simulink model "same_v2"  (R2014b)
settings: Solver=ode45  StartTime=0  StopTime=5  RelTol=1e-3
values from neighbouring files (symbols this model uses):
  a_11 = (a^2*k_1+b^2*k_2)/I_z/u    (= -24.3328872171)    [model.m]
  a_12 = (a*k_1-b*k_2)/I_z    (= 2.49734914361)    [model.m]
  a_21 = (a*k_1-b*k_2)/m/u^2-1    (= -0.900945465806)    [model.m]
  a_22 = (k_1+k_2)/m/u    (= -18.4476774194)    [model.m]
  b_11 = -a*k_1/I_z    (= 50.9018603426)    [model.m]
  b_21 = -k_1/m/u    (= 10.8267096774)    [model.m]
settings Model: Creator=暖的一笔的大学生  LastModifiedBy=暖的一笔的大学生

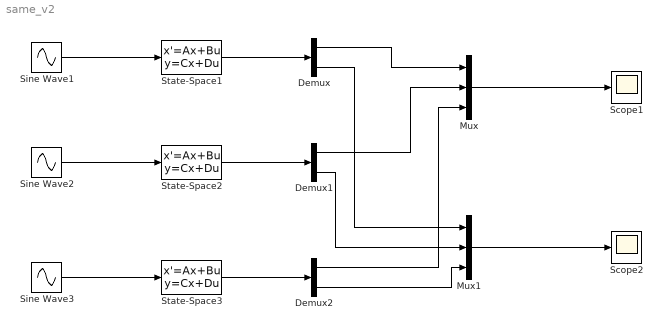
== system same_v2 ==
  Demux : Demux  Outputs=2
  Demux1 : Demux  Outputs=2
  Demux2 : Demux  Outputs=2
  Mux : Mux  Inputs=3
  Mux1 : Mux  Inputs=3
  Scope1 : Scope
  Scope2 : Scope
  Sine Wave1 : Sin  Amplitude=pi/4  SampleTime=0
  Sine Wave2 : Sin  Amplitude=5*pi/22  SampleTime=0
  Sine Wave3 : Sin  Amplitude=5*pi/24  SampleTime=0
  State-Space1 : StateSpace  A=[a_11,a_12;a_21,a_22]  B=[b_11;b_21]  C=[1,0;0,1]  D=[0;0]  X0=[0;0]
  State-Space2 : StateSpace  A=[a_11,a_12;a_21,a_22]  B=[b_11;b_21]  C=[1,0;0,1]  D=[0;0]  X0=[0;0]
  State-Space3 : StateSpace  A=[a_11,a_12;a_21,a_22]  B=[b_11;b_21]  C=[1,0;0,1]  D=[0;0]  X0=[0;0]
  wires:
  Sine Wave2/1 -> State-Space2/1
  Sine Wave3/1 -> State-Space3/1
  State-Space2/1 -> Demux1/1
  State-Space1/1 -> Demux/1
  State-Space3/1 -> Demux2/1
  Demux/1 -> Mux/1
  Demux/2 -> Mux1/1
  Demux1/1 -> Mux/2
  Demux1/2 -> Mux1/2
  Demux2/1 -> Mux/3
  Demux2/2 -> Mux1/3
  Mux/1 -> Scope1/1
  Mux1/1 -> Scope2/1
  Sine Wave1/1 -> State-Space1/1
